simulink library "commdigpbndam2"  (Simulink 5.0)
values from neighbouring files (symbols this model uses):
  i = i + 1    (= 3)    [eyediasi2.m]
undefined symbols (not defined in the file or in its folder): D
libraries: commblksprivate x12, dspsigattribs x6, commdigbbndam2 x6, dspsigops x3
settings Model: RequirementInfo=9  CovMetricSettings=d  Creator=tdelve  LastModifiedBy=mmclerno

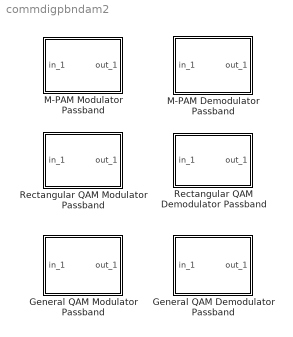
== system commdigpbndam2 ==
  General QAM Demodulator Passband : Subsystem  mask(General QAM Demodulator Passband){SigCon=[exp(2*pi*i*[0:6]/7)], td=1/100, numSamp=1, Fc=3000, Ph=0, InSamp=1/8000}
      mask prompts: SigCon "Signal constellation:"; td "Symbol period (s):"; numSamp "Baseband samples per symbol:"; Fc "Carrier frequency (Hz):"; Ph "Carrier initial phase (rad):"; InSamp "Input sample time (s):"
      mask help:
      | Demodulate the input signal using the quadrature amplitude modulation method.
      |
      | The input signal must be a sample-based scalar.
      mask Help: helpview(commbhelp)
      mask Display:
      | plot(0,0,100,100,[5+1.5*[[0:.8:10] [10:1.6:20] [20:.8:30]] 50 50 50 50+15*[0 1 1 2 2 3]],[85+10*[sin([0:.8:10]*pi*2/5) sin([10:1.6:20]*pi/5) sin([20:.8:30]*pi*2/5)] 85 99 75 85+8*[1 1 -1 -1 1 1]]);
      | disp('\nGeneral\nQAM')
  General QAM Modulator Passband : Subsystem  mask(General QAM Modulator Passband){SigCon=[exp(2*pi*i*[0:6]/7)], td=1/100, numSamp=1, Fc=3000, Ph=0, OutSamp=1/8000}
      mask prompts: SigCon "Signal constellation:"; td "Symbol period (s):"; numSamp "Baseband samples per symbol:"; Fc "Carrier frequency (Hz):"; Ph "Carrier initial phase (rad):"; OutSamp "Output sample time (s):"
      mask help:
      | Modulate the input signal using the quadrature amplitude modulation method.
      |
      | The block only accepts integers as input. The input signal must be a sample-based scalar.
      |
      | The input sample time must equal the symbol period.
      mask Help: helpview(commbhelp)
      mask Display:
      | plot(0,0,100,100,[5+15*[0 1 1 2 2 3] 50 50 50 50+1.5*[[0:.8:10] [10:1.6:20] [20:.8:30]]],[85+8*[1 1 -1 -1 1 1] 85 99 75 85+10*[sin([0:.8:10]*pi*2/5) sin([10:1.6:20]*pi/5) sin([20:.8:30]*pi*2/5)]]);
      | disp('\nGeneral\nQAM')
  M-PAM Demodulator Passband : Subsystem  mask(M-PAM Demodulator Passband){M=4, OutType=Integer, Dec=Binary, PowType=Min. distance between symbols, MinDist=2, AvgPow=1, PeakPow=1, td=1/100, numSamp=1, Fc=3000, Ph=0, InSamp=1/8000}
      mask prompts: M "M-ary number:"; OutType "Output type:"; Dec "Constellation ordering:"; PowType "Normalization method:"; MinDist "Minimum distance:"; AvgPow "Average power (watts):"; PeakPow "Peak power (watts):"; td "Symbol period (s):"; numSamp "Baseband samples per symbol:"; Fc "Carrier frequency (Hz):"; Ph "Carrier initial phase (rad):"; InSamp "Input sample time (s):"
      mask help:
      | Demodulate the input signal using the pulse amplitude modulation method. The M-ary number value must be an even integer.
      |
      | The input signal must be a sample-based scalar. In case of bit output, the width of the output is the number of bits per symbol. The symbols can be either binary-demapped or Gray-demapped into bits.
      mask init:
      | commblkdyampmdemod('M-PAM Demodulator Baseband','update');
      | commblkpbndpammod(gcb,'init');
      mask Help: helpview(commbhelp)
      mask StyleString: edit,popup(Bit|Integer),popup(Binary|Gray),popup(Min. distance between symbols|Average Power|Peak Power),edit,edit,edit,edit,edit,edit,edit,edit
      mask CallbackString: |commblkpbndpammod(gcb,'InType');||commblkpbndpammod(gcb,'PowType');||||||||
      mask Display:
      | plot(0,0,100,100,[5+1.5*[[0:.8:10] [10:1.6:20] [20:.8:30]] 50 50 50 50+15*[0 1 1 2 2 3]],[85+10*[sin([0:.8:10]*pi*2/5) sin([10:1.6:20]*pi/5) sin([20:.8:30]*pi*2/5)] 85 99 75 85+8*[1 1 -1 -1 1 1]]);
      | disp('M-PAM');
  M-PAM Modulator Passband : Subsystem  mask(M-PAM Modulator Passband){M=4, InType=Integer, Enc=Binary, PowType=Min. distance between symbols, MinDist=2, AvgPow=1, PeakPow=1, td=1/100, numSamp=1, Fc=3000, Ph=0, OutSamp=1/8000}
      mask prompts: M "M-ary number:"; InType "Input type:"; Enc "Constellation ordering:"; PowType "Normalization method:"; MinDist "Minimum distance:"; AvgPow "Average power (watts):"; PeakPow "Peak power (watts):"; td "Symbol period (s):"; numSamp "Baseband samples per symbol:"; Fc "Carrier frequency (Hz):"; Ph "Carrier initial phase (rad):"; OutSamp "Output sample time (s):"
      mask help:
      | Modulate the input signal using the pulse amplitude modulation method.
      | The M-ary number value must be an even integer.
      |
      | The input signal must be sample-based. In case of integer input, the input must be a scalar. In case of bit input, the width of the input must equal the number of bits per symbol. The bits can be either binary-mapped or Gray-mapped into symbols.
      |
      | The input sample time must equal the symbol period.
      mask init:
      | commblkdyampmmod('M-PAM Modulator Baseband','update');
      | commblkpbndpammod(gcb,'init');
      mask Help: helpview(commbhelp)
      mask StyleString: edit,popup(Bit|Integer),popup(Binary|Gray),popup(Min. distance between symbols|Average Power|Peak Power),edit,edit,edit,edit,edit,edit,edit,edit
      mask CallbackString: |commblkpbndpammod(gcb,'InType');||commblkpbndpammod(gcb,'PowType');||||||||
      mask Display:
      | plot(0,0,100,100,[5+15*[0 1 1 2 2 3] 50 50 50 50+1.5*[[0:.8:10] [10:1.6:20] [20:.8:30]]],[85+8*[1 1 -1 -1 1 1] 85 99 75 85+10*[sin([0:.8:10]*pi*2/5) sin([10:1.6:20]*pi/5) sin([20:.8:30]*pi*2/5)]]);
      | disp('M-PAM')
  Rectangular QAM Demodulator Passband : Subsystem  mask(Rectangular QAM Demodulator Passband){M=16, OutType=Integer, Dec=Binary, PowType=Min. distance between symbols, MinDist=2, AvgPow=1, PeakPow=1, td=1/100, numSamp=1, Fc=3000, Ph=0, InSamp=1/8000}
      mask prompts: M "M-ary number:"; OutType "Output type:"; Dec "Constellation ordering:"; PowType "Normalization method:"; MinDist "Minimum distance:"; AvgPow "Average power (watts):"; PeakPow "Peak power (watts):"; td "Symbol period (s):"; numSamp "Baseband samples per symbol:"; Fc "Carrier frequency (Hz):"; Ph "Carrier initial phase (rad):"; InSamp "Input sample time (s):"
      mask help:
      | Demodulate the input signal using the rectangular quadrature amplitude modulation method.
      | The M-ary number value needs to be an integer power of two.
      |
      | The input signal must be a sample-based scalar. In case of bit output, the width of the output is the number of bits per symbol. The symbols can be either binary-demapped or Gray-demapped into bits.
      mask init:
      | commblkdyampmdemod('Rectangular QAM Demodulator Baseband','update');
      | commblkpbndqammod(gcb,'init');
      mask Help: helpview(commbhelp)
      mask StyleString: edit,popup(Bit|Integer),popup(Binary|Gray),popup(Min. distance between symbols|Average Power|Peak Power),edit,edit,edit,edit,edit,edit,edit,edit
      mask CallbackString: |commblkpbndqammod(gcb,'InType');||commblkpbndqammod(gcb,'PowType');||||||||
      mask Display:
      | plot(0,0,100,100,[5+1.5*[[0:.8:10] [10:1.6:20] [20:.8:30]] 50 50 50 50+15*[0 1 1 2 2 3]],[85+10*[sin([0:.8:10]*pi*2/5) sin([10:1.6:20]*pi/5) sin([20:.8:30]*pi*2/5)] 85 99 75 85+8*[1 1 -1 -1 1 1]]);
      | disp('\nRectangular\nQAM')
  Rectangular QAM Modulator Passband : Subsystem  mask(Rectangular QAM Modulator Passband){M=16, InType=Integer, Enc=Binary, PowType=Min. distance between symbols, MinDist=2, AvgPow=1, PeakPow=1, td=1/100, numSamp=1, Fc=3000, Ph=0, OutSamp=1/8000}
      mask prompts: M "M-ary number:"; InType "Input type:"; Enc "Constellation ordering:"; PowType "Normalization method:"; MinDist "Minimum distance:"; AvgPow "Average power (watts):"; PeakPow "Peak power (watts):"; td "Symbol period (s):"; numSamp "Baseband samples per symbol:"; Fc "Carrier frequency (Hz):"; Ph "Carrier initial phase (rad):"; OutSamp "Output sample time (s):"
      mask help:
      | Modulate the input signal using the rectangular quadrature amplitude modulation method.
      | The M-ary number value must be an integer power of two.
      |
      | The input signal must be sample-based. In case of integer input, the input must be a scalar. In case of bit input, the width of the input must equal the number of bits per symbol. The bits can be either binary-mapped or Gray-mapped into symbols.
      |
      | The input sample time must equal the symbol period.
      mask init:
      | commblkdyampmmod('Rectangular QAM Modulator Baseband','update');
      | commblkpbndqammod(gcb,'init');
      mask Help: helpview(commbhelp)
      mask StyleString: edit,popup(Bit|Integer),popup(Binary|Gray),popup(Min. distance between symbols|Average Power|Peak Power),edit,edit,edit,edit,edit,edit,edit,edit
      mask CallbackString: |commblkpbndqammod(gcb,'InType');||commblkpbndqammod(gcb,'PowType');||||||||
      mask Display:
      | plot(0,0,100,100,[5+15*[0 1 1 2 2 3] 50 50 50 50+1.5*[[0:.8:10] [10:1.6:20] [20:.8:30]]],[85+8*[1 1 -1 -1 1 1] 85 99 75 85+10*[sin([0:.8:10]*pi*2/5) sin([10:1.6:20]*pi/5) sin([20:.8:30]*pi*2/5)]]);
      | disp('\nRectangular\nQAM')

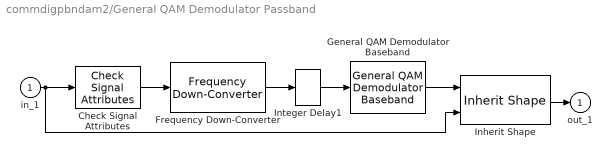
== system commdigpbndam2/General QAM Demodulator Passband ==
  in_1 : Inport
  Check Signal Attributes : dspsigattribs/Check Signal Attributes  SigAttribCheckMethod=Matches attributes exactly  Complexity=Ignore  Frame=Frame-based  DimsCheckMethod=Ignore  Dimensions=1-D  DatatypeCheckMethod=Ignore  DatatypeGeneral=Boolean  DtypeFloatSpecific=Any floating-point  DtypeFixedSpecific=Any fixed-point  DtypeIntSpecific=Any integer  SampleMode=Ignore
  Frequency Down-Converter : commblksprivate/Frequency Down-Converter  Fc=Fc  Ph=Ph  Tin=InSamp  Tout=td/numSamp
  General QAM Demodulator Baseband : commdigbbndam2/General QAM Demodulator Baseband  SigCon=SigCon  numSamp=numSamp
  Inherit Shape : commblksprivate/Inherit Shape
  Integer Delay1 : dspsigops/Integer Delay  delay=numSamp-1  ic=0
  out_1 : Outport  InitialOutput=0
  wires:
  in_1/1 -> Check Signal Attributes/1, Inherit Shape/2
  Check Signal Attributes/1 -> Frequency Down-Converter/1
  Frequency Down-Converter/1 -> Integer Delay1/1
  Integer Delay1/1 -> General QAM Demodulator Baseband/1
  General QAM Demodulator Baseband/1 -> Inherit Shape/1
  Inherit Shape/1 -> out_1/1

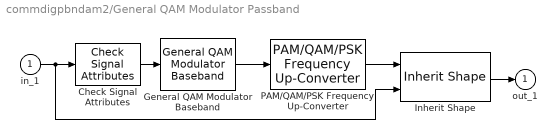
== system commdigpbndam2/General QAM Modulator Passband ==
  in_1 : Inport
  Check Signal Attributes : dspsigattribs/Check Signal Attributes  SigAttribCheckMethod=Matches attributes exactly  Complexity=Ignore  Frame=Frame-based  DimsCheckMethod=Ignore  Dimensions=1-D  DatatypeCheckMethod=Ignore  DatatypeGeneral=Boolean  DtypeFloatSpecific=Any floating-point  DtypeFixedSpecific=Any fixed-point  DtypeIntSpecific=Any integer  SampleMode=Ignore
  General QAM Modulator Baseband : commdigbbndam2/General QAM Modulator Baseband  SigCon=SigCon  numSamp=numSamp
  Inherit Shape : commblksprivate/Inherit Shape
  PAM/QAM/PSK Frequency Up-Converter : commblksprivate/PAM//QAM//PSK Frequency Up-Converter  Fc=Fc  Ph=Ph  Tin=td/numSamp  Tout=OutSamp
  out_1 : Outport  InitialOutput=0
  wires:
  in_1/1 -> Check Signal Attributes/1, Inherit Shape/2
  Check Signal Attributes/1 -> General QAM Modulator Baseband/1
  General QAM Modulator Baseband/1 -> PAM/QAM/PSK Frequency Up-Converter/1
  PAM/QAM/PSK Frequency Up-Converter/1 -> Inherit Shape/1
  Inherit Shape/1 -> out_1/1

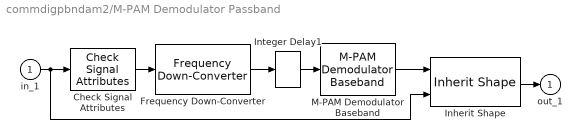
== system commdigpbndam2/M-PAM Demodulator Passband ==
  in_1 : Inport
  Check Signal Attributes : dspsigattribs/Check Signal Attributes  SigAttribCheckMethod=Matches attributes exactly  Complexity=Ignore  Frame=Frame-based  DimsCheckMethod=Ignore  Dimensions=1-D  DatatypeCheckMethod=Ignore  DatatypeGeneral=Boolean  DtypeFloatSpecific=Any floating-point  DtypeFixedSpecific=Any fixed-point  DtypeIntSpecific=Any integer  SampleMode=Ignore
  Frequency Down-Converter : commblksprivate/Frequency Down-Converter  Fc=Fc  Ph=Ph  Tin=InSamp  Tout=td/numSamp
  Inherit Shape : commblksprivate/Inherit Shape
  Integer Delay1 : dspsigops/Integer Delay  delay=numSamp-1  ic=0
  M-PAM Demodulator Baseband : commdigbbndam2/M-PAM Demodulator Baseband  M=M  OutType=Integer  Dec=Binary  PowType=Min. distance between symbols  MinDist=MinDist  AvgPow=AvgPow  PeakPow=PeakPow  numSamp=numSamp
  out_1 : Outport  InitialOutput=0
  wires:
  in_1/1 -> Check Signal Attributes/1, Inherit Shape/2
  M-PAM Demodulator Baseband/1 -> Inherit Shape/1
  Frequency Down-Converter/1 -> Integer Delay1/1
  Integer Delay1/1 -> M-PAM Demodulator Baseband/1
  Check Signal Attributes/1 -> Frequency Down-Converter/1
  Inherit Shape/1 -> out_1/1

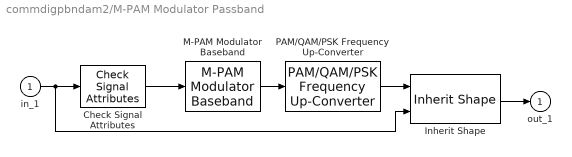
== system commdigpbndam2/M-PAM Modulator Passband ==
  in_1 : Inport
  Check Signal Attributes : dspsigattribs/Check Signal Attributes  SigAttribCheckMethod=Matches attributes exactly  Complexity=Ignore  Frame=Frame-based  DimsCheckMethod=Ignore  Dimensions=1-D  DatatypeCheckMethod=Ignore  DatatypeGeneral=Boolean  DtypeFloatSpecific=Any floating-point  DtypeFixedSpecific=Any fixed-point  DtypeIntSpecific=Any integer  SampleMode=Ignore
  Inherit Shape : commblksprivate/Inherit Shape
  M-PAM Modulator Baseband : commdigbbndam2/M-PAM Modulator Baseband  M=M  InType=Integer  Enc=Binary  PowType=Min. distance between symbols  MinDist=MinDist  AvgPow=AvgPow  PeakPow=PeakPow  numSamp=numSamp
  PAM/QAM/PSK Frequency Up-Converter : commblksprivate/PAM//QAM//PSK Frequency Up-Converter  Fc=Fc  Ph=Ph  Tin=td/numSamp  Tout=OutSamp
  out_1 : Outport  InitialOutput=0
  wires:
  in_1/1 -> Check Signal Attributes/1, Inherit Shape/2
  Check Signal Attributes/1 -> M-PAM Modulator Baseband/1
  M-PAM Modulator Baseband/1 -> PAM/QAM/PSK Frequency Up-Converter/1
  PAM/QAM/PSK Frequency Up-Converter/1 -> Inherit Shape/1
  Inherit Shape/1 -> out_1/1

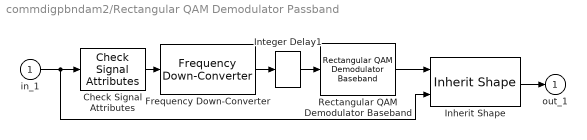
== system commdigpbndam2/Rectangular QAM Demodulator Passband ==
  in_1 : Inport
  Check Signal Attributes : dspsigattribs/Check Signal Attributes  SigAttribCheckMethod=Matches attributes exactly  Complexity=Ignore  Frame=Frame-based  DimsCheckMethod=Ignore  Dimensions=1-D  DatatypeCheckMethod=Ignore  DatatypeGeneral=Boolean  DtypeFloatSpecific=Any floating-point  DtypeFixedSpecific=Any fixed-point  DtypeIntSpecific=Any integer  SampleMode=Ignore
  Frequency Down-Converter : commblksprivate/Frequency Down-Converter  Fc=Fc  Ph=Ph  Tin=InSamp  Tout=td/numSamp
  Inherit Shape : commblksprivate/Inherit Shape
  Integer Delay1 : dspsigops/Integer Delay  delay=numSamp-1  ic=0
  Rectangular QAM Demodulator Baseband : commdigbbndam2/Rectangular QAM Demodulator Baseband  M=M  OutType=Integer  Dec=Binary  PowType=Min. distance between symbols  MinDist=MinDist  AvgPow=AvgPow  PeakPow=PeakPow  Ph=0  numSamp=numSamp
  out_1 : Outport  InitialOutput=0
  wires:
  in_1/1 -> Check Signal Attributes/1, Inherit Shape/2
  Check Signal Attributes/1 -> Frequency Down-Converter/1
  Frequency Down-Converter/1 -> Integer Delay1/1
  Integer Delay1/1 -> Rectangular QAM Demodulator Baseband/1
  Rectangular QAM Demodulator Baseband/1 -> Inherit Shape/1
  Inherit Shape/1 -> out_1/1

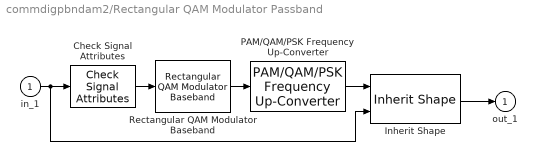
== system commdigpbndam2/Rectangular QAM Modulator Passband ==
  in_1 : Inport
  Check Signal Attributes : dspsigattribs/Check Signal Attributes  SigAttribCheckMethod=Matches attributes exactly  Complexity=Ignore  Frame=Frame-based  DimsCheckMethod=Ignore  Dimensions=1-D  DatatypeCheckMethod=Ignore  DatatypeGeneral=Boolean  DtypeFloatSpecific=Any floating-point  DtypeFixedSpecific=Any fixed-point  DtypeIntSpecific=Any integer  SampleMode=Ignore
  Inherit Shape : commblksprivate/Inherit Shape
  PAM/QAM/PSK Frequency Up-Converter : commblksprivate/PAM//QAM//PSK Frequency Up-Converter  Fc=Fc  Ph=Ph  Tin=td/numSamp  Tout=OutSamp
  Rectangular QAM Modulator Baseband : commdigbbndam2/Rectangular QAM Modulator Baseband  M=M  InType=Integer  Enc=Binary  PowType=Min. distance between symbols  MinDist=MinDist  AvgPow=AvgPow  PeakPow=PeakPow  Ph=0  numSamp=numSamp
  out_1 : Outport  InitialOutput=0
  wires:
  in_1/1 -> Check Signal Attributes/1, Inherit Shape/2
  Check Signal Attributes/1 -> Rectangular QAM Modulator Baseband/1
  Rectangular QAM Modulator Baseband/1 -> PAM/QAM/PSK Frequency Up-Converter/1
  PAM/QAM/PSK Frequency Up-Converter/1 -> Inherit Shape/1
  Inherit Shape/1 -> out_1/1
